simulink model "single_cell_battery_pre_thermal_frozen"  (R2025b)
settings: Solver=FixedStepDiscrete  StartTime=0.0  StopTime=1400  FixedStep=0.1  RelTol=1e-3
values from neighbouring files (symbols this model uses):
  OCV_2d = [3.15119810709 3.1633525458 3.1755069845 3.1876614232 3.19981586191 3.21197030061 3.22412473931 3.23627917802 3.24843361672 3.26058805543 3.27274249413 3.28489693283 ... (303 elements, 101x3)]    [params_all_temps_final.mat]
  Q_nom = 2.9    [ocv_lookup_25C.mat]    (also in params_0C_final.mat = 2.995; params_25C_final.mat = 2.995; params_all_temps_final.mat = 2.995)
  soc_common = [0.17 0.245454545455 0.320909090909 0.396363636364 0.471818181818 0.547272727273 0.622727272727 0.698181818182 0.773636363636 0.849090909091 0.924545454545 1]    [params_all_temps_final.mat]
  soc_ocv_common = [0 0.01 0.02 0.03 0.04 0.05 0.06 0.07 0.08 0.09 0.1 0.11 ... (101 elements, 101x1)]    [params_all_temps_final.mat]
  temp_bp = [0 10 25]    [params_all_temps_final.mat]
  temp_bp_ocv = [0 10 25]    [params_all_temps_final.mat]
  Ts = 0.1    [ocv_lookup_25C.mat]    (also in params_0C_final.mat; params_25C_final.mat; params_all_temps_final.mat)
undefined symbols (not defined in the file or in its folder): C1, C2, DiscIntNeverNeededParam, I_test, inv_C1_2d_fixed, neg_inv_R1C1_2d_fixed, R0, R0_2d_fix, R1, R2, SoC_init, T_cell
settings Model: PacingRate=0.890000  Creator=mahad  LastModifiedBy=mahad
settings DataIOCC: SignalLogging=off  SaveTime=off
settings DebuggingCC: ReadBeforeWriteMsg=DisableAll  WriteAfterWriteMsg=DisableAll  WriteAfterReadMsg=DisableAll  MultiTaskDSMMsg=none
settings ModelReferenceCC: UpdateModelReferenceTargets=IfOutOfDate
settings SFSimCC: SFSimEcho=off

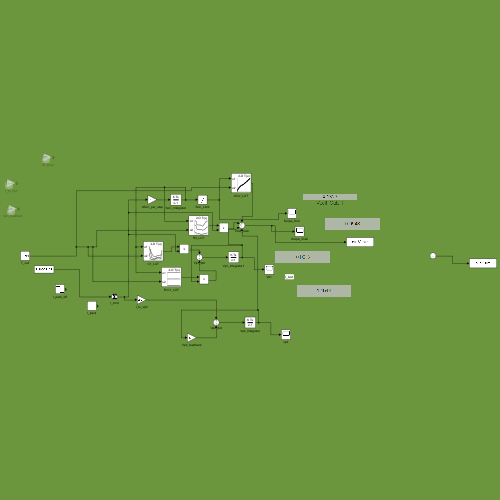
[thumbnail: Simulink's stored preview of the top-level diagram]
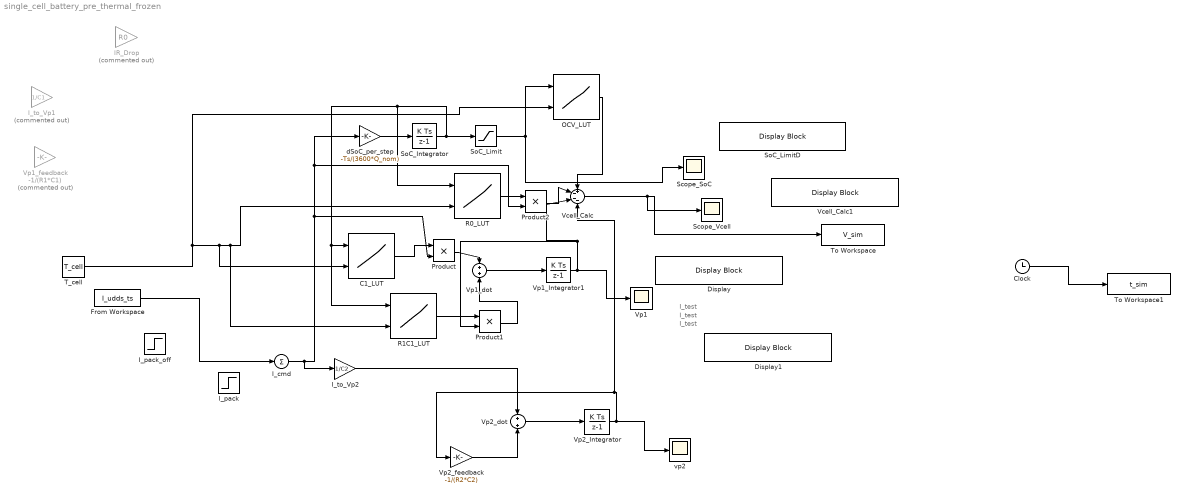
== system single_cell_battery_pre_thermal_frozen ==
  note: I_test
  note: I_test
  note: I_test
  C1_LUT : Lookup_n-D  BreakpointsForDimension1=soc_common  BreakpointsForDimension2=temp_bp  Table=inv_C1_2d_fixed  ExtrapMethod=Clip  InternalRulePriority=Speed  RndMeth=Simplest
      settings: InputPortMap=u0,u1
  Clock : Clock
  Display : DisplayBlock  LabelPosition=Hide  Transparency=1  GridColor=[0.502, 0.502, 0.502]
  Display1 : DisplayBlock  LabelPosition=Hide  Transparency=1  GridColor=[0.502, 0.502, 0.502]
  From Workspace : FromWorkspace  VariableName=I_udds_ts
  IR_Drop : Gain  Commented=on  Gain=R0
  I_cmd : Sum  Inputs=+
  I_pack : Step  Time=0  After=I_test  SampleTime=0.1
  I_pack_off : Step  Time=10  After=-I_test  SampleTime=0.1
  I_to_Vp1 : Gain  Commented=on  Gain=1/C1
  I_to_Vp2 : Gain  Gain=1/C2
  OCV_LUT : Lookup_n-D  BreakpointsForDimension1=soc_ocv_common  BreakpointsForDimension2=temp_bp_ocv  BeginIndexSearchUsingPreviousIndexResult=on  Table=OCV_2d  ExtrapMethod=Clip  InternalRulePriority=Speed  RndMeth=Simplest
      settings: InputPortMap=u0,u1
  Product : Product
  Product1 : Product
  Product2 : Product
  R0_LUT : Lookup_n-D  BreakpointsForDimension1=soc_common  BreakpointsForDimension2=temp_bp  Table=R0_2d_fix  ExtrapMethod=Clip  InternalRulePriority=Speed  RndMeth=Simplest
      settings: InputPortMap=u0,u1
  R1C1_LUT : Lookup_n-D  BreakpointsForDimension1=soc_common  BreakpointsForDimension2=temp_bp  Table=neg_inv_R1C1_2d_fixed  ExtrapMethod=Clip  InternalRulePriority=Speed  RndMeth=Simplest
      settings: InputPortMap=u0,u1
  Scope_SoC : Scope
      settings: ActiveDisplayYMinimum=0.99409967767112239  ActiveDisplayYMaximum=1.0006555913698754  DataLoggingVariableName=SoC_log
  Scope_Vcell : Scope
      settings: ActiveDisplayYMinimum=3.9024724539871976  ActiveDisplayYMaximum=4.18640131557632
  SoC_Integrator : DiscreteIntegrator  InitialCondition=SoC_init  SampleTime=0.1  ICPrevOutput=DiscIntNeverNeededParam  ICPrevScaledInput=DiscIntNeverNeededParam
  SoC_Limit : Saturate  UpperLimit=1  LowerLimit=0
  SoC_LimitD : DisplayBlock  LabelPosition=Bottom  Transparency=1  GridColor=[0.502, 0.502, 0.502]
  T_cell : Constant  Value=T_cell  SampleTime=-1
  To Workspace : ToWorkspace  VariableName=V_sim  SampleTime=-1
  To Workspace1 : ToWorkspace  VariableName=t_sim  SampleTime=-1
  Vcell_Calc : Sum  Inputs=+---
  Vcell_Calc1 : DisplayBlock  LabelPosition=Hide  Transparency=1  GridColor=[0.502, 0.502, 0.502]
  Vp1 : Scope
      settings: ActiveDisplayYMinimum=-0.0028893234136200406  ActiveDisplayYMaximum=0.026003910722580369  DataLoggingVariableName=ScopeData2
  Vp1_Integrator1 : DiscreteIntegrator  SampleTime=0.1  ICPrevOutput=DiscIntNeverNeededParam  ICPrevScaledInput=DiscIntNeverNeededParam
  Vp1_dot : Sum
  Vp1_feedback : Gain  Commented=on  Gain=-1/(R1*C1)
  Vp2_Integrator : DiscreteIntegrator  SampleTime=0.1  ICPrevOutput=DiscIntNeverNeededParam  ICPrevScaledInput=DiscIntNeverNeededParam
  Vp2_dot : Sum
  Vp2_feedback : Gain  Gain=-1/(R2*C2)
  dSoC_per_step : Gain  Gain=-Ts/(3600*Q_nom)
  vp2 : Scope
      settings: ActiveDisplayYMinimum=-0.00021306760205067724  ActiveDisplayYMaximum=0.0019176084184560956  DataLoggingVariableName=ScopeData3
  wires:
  dSoC_per_step/1 -> SoC_Integrator/1
  SoC_Integrator/1 -> R1C1_LUT/1, C1_LUT/1, R0_LUT/1, SoC_Limit/1
  SoC_Limit/1 -> OCV_LUT/1, Scope_SoC/1
  OCV_LUT/1 -> Vcell_Calc/1
  Vcell_Calc/1 -> To Workspace/1, Scope_Vcell/1
  Vp1_Integrator1/1 -> Vp1/1, Product1/2, Vcell_Calc/3
  Vp1_dot/1 -> Vp1_Integrator1/1
  Vp2_dot/1 -> Vp2_Integrator/1
  Vp2_Integrator/1 -> vp2/1, Vcell_Calc/4, Vp2_feedback/1
  I_to_Vp2/1 -> Vp2_dot/1
  Vp2_feedback/1 -> Vp2_dot/2
  I_cmd/1 -> I_to_Vp2/1, Product2/2, dSoC_per_step/1, Product/2
  Clock/1 -> To Workspace1/1
  C1_LUT/1 -> Product/1
  Product/1 -> Vp1_dot/1
  R1C1_LUT/1 -> Product1/1
  Product1/1 -> Vp1_dot/2
  T_cell/1 -> OCV_LUT/2, C1_LUT/2, R1C1_LUT/2, R0_LUT/2
  R0_LUT/1 -> Product2/1
  Product2/1 -> Vcell_Calc/2
  From Workspace/1 -> I_cmd/1
